simulink model "SimulinkLR1"  (R2016a)
settings: Solver=VariableStepAuto  StartTime=0.0  StopTime=10.0  RelTol=1e-3
values from neighbouring files (symbols this model uses):
  alpha = alpha1    (= 0.2)    [LR1_KGP.m]    (also in LR1_NKGP.m = 0.01)
  f0 = 1200    [LR1_KGP.m]    (also in LR1_NKGP.m; Untitled.m = 1.2)
  N = 1000    [LR1_KGP.m]    (also in LR1_NKGP.m)
  T = sum( (noise+u).*u )    [LR1_KGP.m]    (also in LR1_NKGP.m = 0.012; Untitled.m = 12)
  Variance = Disp(i)    [LR1_KGP.m]
undefined symbols (not defined in the file or in its folder): DiscIntNeverNeededParam, erfcinv
libraries: dspsrcs4 x1
settings Model: Creator=Энверыч  LastModifiedBy=Энверыч

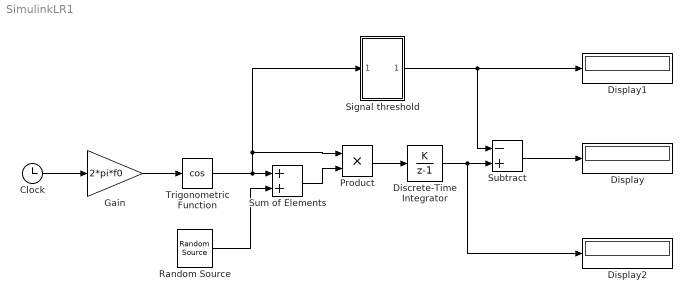
== system SimulinkLR1 ==
  Clock : Clock
  Discrete-Time Integrator : DiscreteIntegrator  IntegratorMethod=Accumulation: Forward Euler  InitialConditionSetting=State (most efficient)  SampleTime=T/N  ICPrevOutput=DiscIntNeverNeededParam  ICPrevScaledInput=DiscIntNeverNeededParam
  Display : Display
  Display1 : Display
  Display2 : Display
  Gain : Gain  Gain=2*pi*f0
  Product : Product
  Random Source : dspsrcs4/Random Source  SrcType=Uniform  NormMethod=Ziggurat  CltLength=12  MinVal=0  MaxVal=1  MeanVal=0  VarVal=1  RepMode=Not repeatable  rawSeed=1  IsInherit=off  SampMode=Discrete  SampTime=T/N  SampFrame=1  DataType=Double  OutComplex=Real  OutputFrames=off
  Signal threshold : Subsystem
  Subtract : Sum  Inputs=-+
  Sum of Elements : Sum
  Trigonometric Function : Trigonometry  Operator=cos
  wires:
  Gain/1 -> Trigonometric Function/1
  Clock/1 -> Gain/1
  Random Source/1 -> Sum of Elements/2
  Product/1 -> Discrete-Time Integrator/1
  Subtract/1 -> Display/1
  Discrete-Time Integrator/1 -> Display2/1, Subtract/2
  Sum of Elements/1 -> Product/2
  Trigonometric Function/1 -> Product/1, Signal threshold/1(In1), Sum of Elements/1
  Signal threshold/1(Out1) -> Display1/1, Subtract/1

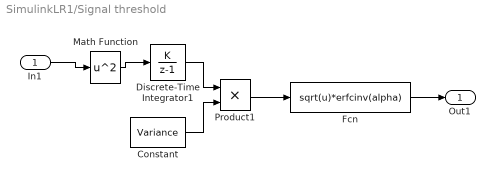
== system SimulinkLR1/Signal threshold ==
  In1 : Inport
  Constant : Constant  Value=Variance
  Discrete-Time Integrator1 : DiscreteIntegrator  IntegratorMethod=Accumulation: Forward Euler  InitialConditionSetting=State (most efficient)  SampleTime=T/N  ICPrevOutput=DiscIntNeverNeededParam  ICPrevScaledInput=DiscIntNeverNeededParam
  Fcn : Fcn  Expr=sqrt(u)*erfcinv(alpha)
  Math Function : Math  Operator=square  SaturateOnIntegerOverflow=on
  Product1 : Product
  Out1 : Outport
  wires:
  In1/1 -> Math Function/1
  Fcn/1 -> Out1/1
  Product1/1 -> Fcn/1
  Constant/1 -> Product1/2
  Math Function/1 -> Discrete-Time Integrator1/1
  Discrete-Time Integrator1/1 -> Product1/1
